simulink model "GEOFENCING"  (R2022b)
settings: Solver=VariableStepAuto  StartTime=0.0  StopTime=10.0  RelTol=1e-3
settings Model: Creator=lucaerviati  LastModifiedBy=lucaerviati

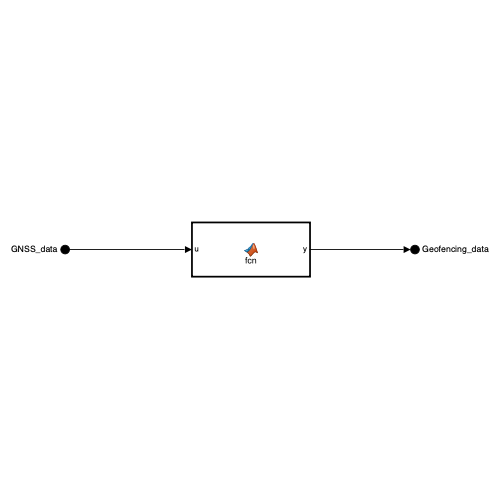
[thumbnail: Simulink's stored preview of the top-level diagram]
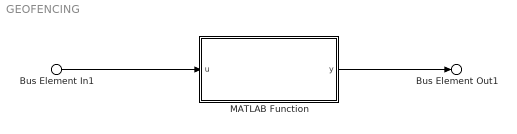
== system GEOFENCING ==
  Bus Element In1 : Inport  PortName=GNSS_data
  MATLAB Function : MATLAB Function  TreatAsAtomicUnit=on
  Bus Element Out1 : Outport  PortName=Geofencing_data
  wires:
  MATLAB Function/1(y) -> Bus Element Out1/1
  Bus Element In1/1 -> MATLAB Function/1(u)

== matlab function GEOFENCING/MATLAB Function ==
  data: u input; y output
function y = fcn(u)
u = [24124,
    24122,
    13143]
y = u;
